simulink library "SUB_ECU_L4_MABX_HW_Interface_PIC_PB"  (R2018a)
settings: Solver=VariableStepAuto  StartTime=0.0  StopTime=10.0  RelTol=1e-3
PostLoadFcn:
  | , if any(exist('dsrtsu_mdlpostloadfcn', 'file') == [2, 3, 6]), try dsrtsu_mdlpostloadfcn('Execute', bdroot); catch fprintf('Error in PostLoadFcn (dsrtsu_mdlpostloadfcn) for model "%s":\n %s\n', bdroot, lasterr); end, end,
undefined symbols (not defined in the file or in its folder): CANR_PROPB_REAX_3_13_CHANNEL_APV, CANR_PROPB_REAX_4_13_CHANNEL_APV, CANR_PROPB_XPR_1_50_CHANNEL_APV, ENUM_CAN_RX_T, ENUM_CAN_TX_T, ENUM_REAX_OPERATION_MODE_T, ENUM_SIGNAL_HEALTH_T, ENUM_XBR_CONTROL_MODE_T, ENUM_XBR_EBI_MODE_T, ENUM_XBR_PASS_THROUGH_ACTIVE_T, ENUM_XBR_PRIORITY_T, ENUM_XPR_INHIBIT_PARK_MANUAL_T, ENUM_XPR_INHIBIT_UNPARK_MANUAL_T, ENUM_XPR_PARK_MANUAL_T, ENUM_XPR_UNPARK_MANUAL_T, PROPB_REAX_1_E4_DES_POS_SIG_SRC_APV, PROPB_REAX_1_E4_DESIRED_OPMODE_APV, PROPB_REAX_1_E4_DESIRED_POSITION_APV, PROPB_REAX_CHANNEL_APV, ptc_matlab_lib
libraries: PTC_MBDS_LIB x293, rtican x158, simulink x61, EmE_MBD_Blockset x38, rti1401lib_dio_type4 x14, simulink_need_slupdate x7, $bdroot x5, rti1401lib_adc_type4 x3, rtmapslib x3, dsa_tcpip_lib x2, SUB_ECU_L4_MABX_HW_Interface_PTC_1571 x1, rtitasklib x1
(part 20 of 49)

== system SUB_ECU_L4_MABX_HW_Interface_PIC_PB/CAN_PIC_PB/CAN_RX_VI_00/Decode_VI ==
  RawData : Inport  OutDataTypeStr=uint8  PortDimensions=17
  Add : Sum  Inputs=+  InputSameDT=on
  Add1 : Sum  Inputs=+  InputSameDT=on
  Bus Creator : BusCreator  Inputs=3
  Compare To Zero1 : simulink/Logic and Bit Operations/Compare To Zero  relop===  OutDataTypeStr=boolean
  Compare To Zero2 : simulink/Logic and Bit Operations/Compare To Zero  relop===  OutDataTypeStr=boolean
  Constant : Constant  Value=false
  Constant1 : Constant  Value=false
  Data Type Conversion{,1..16} (17 alike) : DataTypeConversion  OutDataTypeStr=uint8
  Demux : Demux  Outputs=17
  Logical Operator : Logic  OutDataTypeStr=boolean
  Logical Operator1 : Logic  OutDataTypeStr=boolean
  Mux : Mux  Inputs=17
  Relational Operator1 : RelationalOperator  Operator=~=  OutDataTypeStr=boolean  RndMeth=Nearest  InputSameDT=on
  Relational Operator2 : RelationalOperator  Operator=~=  OutDataTypeStr=boolean  RndMeth=Nearest  InputSameDT=on
  SR flip-flop : EmE_MBD_Blockset/Logic and Bit Operations/SR flip-flop
      settings: SourceProductName=PACCAR EmE MBD Blockset
  SR flip-flop1 : EmE_MBD_Blockset/Logic and Bit Operations/SR flip-flop
      settings: SourceProductName=PACCAR EmE MBD Blockset
  TRUCK_1571_VIN_CPV : Constant  Value=uint8('1XPBDP9XXGD305352')
  TRUCK_166_VIN_CPV : Constant  Value=uint8('1XKYDP9X1EJ388961')
  Unit_Delay{,1..3} (4 alike) : UnitDelay  InitialCondition=true  SampleTime=-1
      settings: AttributesFormatString=IC: %<vinit>
  VI : Outport
  wires:
  RawData/1 -> Demux/1
  Mux/1 -> Relational Operator2/2, Relational Operator1/2, Bus Creator/1  "SPN237_VehicleIdentificationNumber"
  Data Type Conversion16/1 -> Mux/17
  Data Type Conversion5/1 -> Mux/6
  Data Type Conversion/1 -> Mux/1
  Data Type Conversion1/1 -> Mux/2
  Data Type Conversion6/1 -> Mux/7
  Data Type Conversion10/1 -> Mux/11
  Data Type Conversion11/1 -> Mux/12
  Data Type Conversion7/1 -> Mux/8
  Data Type Conversion12/1 -> Mux/13
  Data Type Conversion13/1 -> Mux/15
  Data Type Conversion8/1 -> Mux/9
  Data Type Conversion15/1 -> Mux/16
  Data Type Conversion2/1 -> Mux/3
  Data Type Conversion3/1 -> Mux/4
  Data Type Conversion9/1 -> Mux/10
  Data Type Conversion4/1 -> Mux/5
  Data Type Conversion14/1 -> Mux/14
  Relational Operator1/1 -> Add/1
  Add/1 -> Compare To Zero1/1
  TRUCK_166_VIN_CPV/1 -> Relational Operator2/1
  TRUCK_1571_VIN_CPV/1 -> Relational Operator1/1
  Relational Operator2/1 -> Add1/1
  Add1/1 -> Compare To Zero2/1
  SR flip-flop/1 -> Bus Creator/3  "F_Truck1571_VIN_Match"
  SR flip-flop1/1 -> Bus Creator/2  "F_Truck166_VIN_Match"
  Demux/8 -> Data Type Conversion7/1  "byte7"
  Demux/9 -> Data Type Conversion8/1  "byte8"
  Demux/7 -> Data Type Conversion6/1  "byte6"
  Demux/6 -> Data Type Conversion5/1  "byte5"
  Demux/10 -> Data Type Conversion9/1  "byte9"
  Demux/11 -> Data Type Conversion10/1  "byte10"
  Demux/5 -> Data Type Conversion4/1  "byte4"
  Demux/12 -> Data Type Conversion11/1  "byte11"
  Demux/4 -> Data Type Conversion3/1  "byte3"
  Demux/13 -> Data Type Conversion12/1  "byte12"
  Demux/3 -> Data Type Conversion2/1  "byte2"
  Demux/2 -> Data Type Conversion1/1  "byte1"
  Demux/14 -> Data Type Conversion14/1  "byte13"
  Demux/15 -> Data Type Conversion13/1  "byte14"
  Demux/1 -> Data Type Conversion/1  "byte0"
  Demux/16 -> Data Type Conversion15/1  "byte15"
  Demux/17 -> Data Type Conversion16/1  "byte16"
  Bus Creator/1 -> VI/1  "Signals"
  Unit_Delay/1 -> SR flip-flop/2
  Constant/1 -> Unit_Delay/1
  Compare To Zero1/1 -> Logical Operator/2
  Unit_Delay1/1 -> SR flip-flop1/2
  Constant1/1 -> Unit_Delay1/1
  SR flip-flop1/2 -> Unit_Delay3/1
  Logical Operator/1 -> SR flip-flop/1
  Logical Operator1/1 -> SR flip-flop1/1
  Compare To Zero2/1 -> Logical Operator1/2
  SR flip-flop/2 -> Unit_Delay2/1
  Unit_Delay2/1 -> Logical Operator1/1
  Unit_Delay3/1 -> Logical Operator/1

== system SUB_ECU_L4_MABX_HW_Interface_PIC_PB/CAN_PIC_PB/Decode_PropB_REAX_3/decode_byte1 ==
  byte1 : Inport
  AND1 : PTC_MBDS_LIB/MBDS Standard Library/Basic Operations/Logic and Bit Operations/AND  BitwiseMode=on  Inputs=1  UseBitMask=on  BitMask=bin2dec('11110000')  OutDataTypeStr=uint8  PTC_MBDS_BlockVersion=5.41  PTC_BlockType=PTC_MBDS_AND
      settings: AttributesFormatString=bitwise  SourceProductName=PACCAR Technical Center MBDS Library
  AND2 : PTC_MBDS_LIB/MBDS Standard Library/Basic Operations/Logic and Bit Operations/AND  BitwiseMode=on  Inputs=1  UseBitMask=on  BitMask=bin2dec('00001111')  OutDataTypeStr=uint8  PTC_MBDS_BlockVersion=5.41  PTC_BlockType=PTC_MBDS_AND
      settings: AttributesFormatString=bitwise  SourceProductName=PACCAR Technical Center MBDS Library
  Bus Creator : BusCreator  Inputs=2
  "Shift_Arithmetic " : ArithShift  BitShiftNumber=4
  Out : Outport
  wires:
  "Shift_Arithmetic "/1 -> Bus Creator/2  "PropB_REAX_3_ReqOperatingMode"
  byte1/1 -> AND1/1, AND2/1
  AND2/1 -> Bus Creator/1  "PropB_REAX_3_CurrentOperatingMode"
  AND1/1 -> "Shift_Arithmetic "/1
  Bus Creator/1 -> Out/1

== system SUB_ECU_L4_MABX_HW_Interface_PIC_PB/CAN_PIC_PB/Decode_PropB_REAX_3/decode_byte2 ==
  byte2 : Inport
  Bus Creator : BusCreator  Inputs=1
  Out : Outport
  wires:
  byte2/1 -> Bus Creator/1  "PropB_REAX_3_StatusErrMsg"
  Bus Creator/1 -> Out/1

== system SUB_ECU_L4_MABX_HW_Interface_PIC_PB/CAN_PIC_PB/Decode_PropB_REAX_3/decode_byte3_byte4 ==
  byte3 : Inport
  byte4 : Inport  Port=2
  Bus Creator : BusCreator  Inputs=1
  Constant : Constant  Value=1/1024
  Data Type Conversion1 : DataTypeConversion  OutDataTypeStr=uint16  SaturateOnIntegerOverflow=on
  Data Type Conversion2 : DataTypeConversion  OutDataTypeStr=uint16  SaturateOnIntegerOverflow=on
  Data Type Conversion3 : DataTypeConversion  OutDataTypeStr=int16  ConvertRealWorld=Stored Integer (SI)
  Data Type Conversion4 : DataTypeConversion  SaturateOnIntegerOverflow=on
  OR : PTC_MBDS_LIB/MBDS Standard Library/Basic Operations/Logic and Bit Operations/OR  BitwiseMode=on  Inputs=2  UseBitMask=off  BitMask='A7'  OutDataTypeStr=uint16  PTC_MBDS_BlockVersion=5.41  PTC_BlockType=PTC_MBDS_OR
      settings: AttributesFormatString=bitwise  SourceProductName=PACCAR Technical Center MBDS Library
  Product : Product  Inputs=**  OutDataTypeStr=single  SaturateOnIntegerOverflow=on  InputSameDT=on
      settings: AttributesFormatString=Saturate: %<SaturateOnIntegerOverflow>
  Shift_Arithmetic 1 : ArithShift  BitShiftNumber=-8
  Out : Outport
  wires:
  Product/1 -> Bus Creator/1  "PropB_REAX_3_HandwheelTorque"
  Constant/1 -> Product/2
  Data Type Conversion3/1 -> Data Type Conversion4/1
  byte3/1 -> Data Type Conversion1/1
  byte4/1 -> Data Type Conversion2/1
  Data Type Conversion2/1 -> Shift_Arithmetic 1/1
  Data Type Conversion1/1 -> OR/1
  Shift_Arithmetic 1/1 -> OR/2
  OR/1 -> Data Type Conversion3/1
  Data Type Conversion4/1 -> Product/1
  Bus Creator/1 -> Out/1

== system SUB_ECU_L4_MABX_HW_Interface_PIC_PB/CAN_PIC_PB/Decode_PropB_REAX_3/decode_byte5_byte6 ==
  byte5 : Inport
  byte6 : Inport  Port=2
  Bus Creator : BusCreator  Inputs=1
  Constant1 : Constant  Value=1/1024
  Data Type Conversion1 : DataTypeConversion  SaturateOnIntegerOverflow=on
  Data Type Conversion4 : DataTypeConversion  OutDataTypeStr=uint16  SaturateOnIntegerOverflow=on
  Data Type Conversion5 : DataTypeConversion  OutDataTypeStr=uint16  SaturateOnIntegerOverflow=on
  Data Type Conversion6 : DataTypeConversion  OutDataTypeStr=int16  ConvertRealWorld=Stored Integer (SI)
  OR1 : PTC_MBDS_LIB/MBDS Standard Library/Basic Operations/Logic and Bit Operations/OR  BitwiseMode=on  Inputs=2  UseBitMask=off  BitMask='A7'  OutDataTypeStr=uint16  PTC_MBDS_BlockVersion=5.41  PTC_BlockType=PTC_MBDS_OR
      settings: AttributesFormatString=bitwise  SourceProductName=PACCAR Technical Center MBDS Library
  Product1 : Product  Inputs=**  OutDataTypeStr=single  SaturateOnIntegerOverflow=on  InputSameDT=on
      settings: AttributesFormatString=Saturate: %<SaturateOnIntegerOverflow>
  Shift_Arithmetic 2 : ArithShift  BitShiftNumber=-8
  Out : Outport
  wires:
  byte5/1 -> Data Type Conversion4/1
  byte6/1 -> Data Type Conversion5/1
  Shift_Arithmetic 2/1 -> OR1/2
  Data Type Conversion5/1 -> Shift_Arithmetic 2/1
  Data Type Conversion4/1 -> OR1/1
  OR1/1 -> Data Type Conversion6/1
  Data Type Conversion6/1 -> Data Type Conversion1/1
  Constant1/1 -> Product1/2
  Product1/1 -> Bus Creator/1  "PropB_REAX_3_HandwheelVelocity"
  Data Type Conversion1/1 -> Product1/1
  Bus Creator/1 -> Out/1

== system SUB_ECU_L4_MABX_HW_Interface_PIC_PB/CAN_PIC_PB/Decode_PropB_REAX_3/decode_byte7_byte8 ==
  byte7 : Inport
  byte8 : Inport  Port=2
  Bus Creator : BusCreator  Inputs=1
  Constant2 : Constant  Value=360/8192
  Data Type Conversion1 : DataTypeConversion  SaturateOnIntegerOverflow=on
  Data Type Conversion7 : DataTypeConversion  OutDataTypeStr=uint16  SaturateOnIntegerOverflow=on
  Data Type Conversion8 : DataTypeConversion  OutDataTypeStr=uint16  SaturateOnIntegerOverflow=on
  Data Type Conversion9 : DataTypeConversion  OutDataTypeStr=int16  ConvertRealWorld=Stored Integer (SI)
  OR2 : PTC_MBDS_LIB/MBDS Standard Library/Basic Operations/Logic and Bit Operations/OR  BitwiseMode=on  Inputs=2  UseBitMask=off  BitMask='A7'  OutDataTypeStr=uint16  PTC_MBDS_BlockVersion=5.41  PTC_BlockType=PTC_MBDS_OR
      settings: AttributesFormatString=bitwise  SourceProductName=PACCAR Technical Center MBDS Library
  Product2 : Product  Inputs=**  OutDataTypeStr=single  SaturateOnIntegerOverflow=on  InputSameDT=on
      settings: AttributesFormatString=Saturate: %<SaturateOnIntegerOverflow>
  Shift_Arithmetic 3 : ArithShift  BitShiftNumber=-8
  Out : Outport
  wires:
  byte8/1 -> Data Type Conversion8/1
  Product2/1 -> Bus Creator/1  "PropB_REAX_3_PullCompensation"
  byte7/1 -> Data Type Conversion7/1
  Data Type Conversion8/1 -> Shift_Arithmetic 3/1
  Data Type Conversion7/1 -> OR2/1
  Shift_Arithmetic 3/1 -> OR2/2
  OR2/1 -> Data Type Conversion9/1
  Constant2/1 -> Product2/2
  Data Type Conversion9/1 -> Data Type Conversion1/1
  Data Type Conversion1/1 -> Product2/1
  Bus Creator/1 -> Out/1

== system SUB_ECU_L4_MABX_HW_Interface_PIC_PB/CAN_PIC_PB/Decode_PropB_REAX_4/decode_byte1 ==
  byte1 : Inport
  AND : PTC_MBDS_LIB/MBDS Standard Library/Basic Operations/Logic and Bit Operations/AND  BitwiseMode=on  Inputs=1  UseBitMask=on  BitMask=bin2dec('00000001')  OutDataTypeStr=boolean  PTC_MBDS_BlockVersion=5.41  PTC_BlockType=PTC_MBDS_AND
      settings: AttributesFormatString=bitwise  SourceProductName=PACCAR Technical Center MBDS Library
  AND1 : PTC_MBDS_LIB/MBDS Standard Library/Basic Operations/Logic and Bit Operations/AND  BitwiseMode=on  Inputs=1  UseBitMask=on  BitMask=bin2dec('00000010')  OutDataTypeStr=uint8  PTC_MBDS_BlockVersion=5.41  PTC_BlockType=PTC_MBDS_AND
      settings: AttributesFormatString=bitwise  SourceProductName=PACCAR Technical Center MBDS Library
  AND2 : PTC_MBDS_LIB/MBDS Standard Library/Basic Operations/Logic and Bit Operations/AND  BitwiseMode=on  Inputs=1  UseBitMask=on  BitMask=bin2dec('00000100')  OutDataTypeStr=uint8  PTC_MBDS_BlockVersion=5.41  PTC_BlockType=PTC_MBDS_AND
      settings: AttributesFormatString=bitwise  SourceProductName=PACCAR Technical Center MBDS Library
  Bus Creator : BusCreator  Inputs=3
  Data Type Conversion : DataTypeConversion  OutDataTypeStr=boolean  SaturateOnIntegerOverflow=on
  Data Type Conversion1 : DataTypeConversion  OutDataTypeStr=boolean  SaturateOnIntegerOverflow=on
  "Shift_Arithmetic " : ArithShift  BitShiftNumber=1
  Shift_Arithmetic 1 : ArithShift  BitShiftNumber=2
  Out : Outport
  wires:
  AND/1 -> Bus Creator/1  "PropB_REAX_4_AbsSteeringPosValid"
  AND2/1 -> Shift_Arithmetic 1/1
  byte1/1 -> AND2/1, AND1/1, AND/1
  AND1/1 -> "Shift_Arithmetic "/1
  "Shift_Arithmetic "/1 -> Data Type Conversion/1
  Shift_Arithmetic 1/1 -> Data Type Conversion1/1
  Bus Creator/1 -> Out/1
  Data Type Conversion/1 -> Bus Creator/2  "PropB_REAX_4_PositionIndexValid"
  Data Type Conversion1/1 -> Bus Creator/3  "PropB_REAX_4_DriverControlledEffortsEnabled"

== system SUB_ECU_L4_MABX_HW_Interface_PIC_PB/CAN_PIC_PB/Decode_PropB_REAX_4/decode_byte2 ==
  byte2 : Inport
  Bus Creator : BusCreator  Inputs=1
  SignalConversion : SignalConversion  ConversionOutput=Contiguous copy  OverrideOpt=off
  Out : Outport
  wires:
  byte2/1 -> SignalConversion/1
  SignalConversion/1 -> Bus Creator/1  "PropB_REAX_4_ControlOperatingMode"
  Bus Creator/1 -> Out/1

== system SUB_ECU_L4_MABX_HW_Interface_PIC_PB/CAN_PIC_PB/Decode_PropB_REAX_4/decode_byte3 ==
  byte3 : Inport
  Bus Creator : BusCreator  Inputs=1
  SignalConversion : SignalConversion  ConversionOutput=Contiguous copy  OverrideOpt=off
  Out : Outport
  wires:
  byte3/1 -> SignalConversion/1
  SignalConversion/1 -> Bus Creator/1  "PropB_REAX_4_SystemMode"
  Bus Creator/1 -> Out/1

== system SUB_ECU_L4_MABX_HW_Interface_PIC_PB/CAN_PIC_PB/Decode_PropB_REAX_4/decode_byte5 ==
  byte5 : Inport
  Bus Creator : BusCreator  Inputs=1
  Data Type Conversion4 : DataTypeConversion  OutDataTypeStr=int8  ConvertRealWorld=Stored Integer (SI)
  Data Type Conversion5 : DataTypeConversion  OutDataTypeStr=double  SaturateOnIntegerOverflow=on
  Out : Outport
  wires:
  byte5/1 -> Data Type Conversion4/1
  Data Type Conversion4/1 -> Data Type Conversion5/1
  Data Type Conversion5/1 -> Bus Creator/1  "PropB_REAX_4_PercHandwheelTorque"
  Bus Creator/1 -> Out/1

== system SUB_ECU_L4_MABX_HW_Interface_PIC_PB/CAN_PIC_PB/Decode_PropB_REAX_4/decode_byte6_byte7 ==
  byte6 : Inport
  byte7 : Inport  Port=2
  Bus Creator : BusCreator  Inputs=1
  Data Type Conversion6 : DataTypeConversion  OutDataTypeStr=uint16  SaturateOnIntegerOverflow=on
  Data Type Conversion7 : DataTypeConversion  OutDataTypeStr=uint16  SaturateOnIntegerOverflow=on
  Data Type Conversion8 : DataTypeConversion  OutDataTypeStr=int16  ConvertRealWorld=Stored Integer (SI)
  Data Type Conversion9 : DataTypeConversion  OutDataTypeStr=double  SaturateOnIntegerOverflow=on
  OR : PTC_MBDS_LIB/MBDS Standard Library/Basic Operations/Logic and Bit Operations/OR  BitwiseMode=on  Inputs=2  UseBitMask=off  BitMask='A7'  OutDataTypeStr=uint16  PTC_MBDS_BlockVersion=5.41  PTC_BlockType=PTC_MBDS_OR
      settings: AttributesFormatString=bitwise  SourceProductName=PACCAR Technical Center MBDS Library
  Shift_Arithmetic 2 : ArithShift  BitShiftNumber=-8
  Out : Outport
  wires:
  Data Type Conversion9/1 -> Bus Creator/1  "PropB_REAX_4_AbsSteeringAngle"
  byte6/1 -> Data Type Conversion6/1
  byte7/1 -> Data Type Conversion7/1
  Data Type Conversion6/1 -> OR/1
  Data Type Conversion7/1 -> Shift_Arithmetic 2/1
  Shift_Arithmetic 2/1 -> OR/2
  Data Type Conversion8/1 -> Data Type Conversion9/1
  OR/1 -> Data Type Conversion8/1
  Bus Creator/1 -> Out/1

== system SUB_ECU_L4_MABX_HW_Interface_PIC_PB/CAN_PIC_PB/Decode_PropB_REAX_4/decode_byte8 ==
  byte8 : Inport
  Bus Creator : BusCreator  Inputs=1
  Data Type Conversion10 : DataTypeConversion  OutDataTypeStr=int8  ConvertRealWorld=Stored Integer (SI)
  Data Type Conversion11 : DataTypeConversion  OutDataTypeStr=double  SaturateOnIntegerOverflow=on
  Out : Outport
  wires:
  Data Type Conversion11/1 -> Bus Creator/1  "PropB_REAX_4_PercMotorTorque"
  Data Type Conversion10/1 -> Data Type Conversion11/1
  byte8/1 -> Data Type Conversion10/1
  Bus Creator/1 -> Out/1

== system SUB_ECU_L4_MABX_HW_Interface_PIC_PB/DIGITAL/Debounce/On Delay ==
  In : Inport
  time_ms : Inport  Port=2
  AND : Logic  IconShape=distinctive  AllPortsSameDT=off  OutDataTypeStr=boolean
  Compare To Zero : simulink/Logic and Bit Operations/Compare To Zero  relop=>  OutDataTypeStr=boolean
  Constant0 : Constant  Value=0
  Constant1 : Constant
  Gain : Gain  Gain=0.1
  LessThanOrEqual : RelationalOperator  Operator=<=  OutDataTypeStr=boolean  RndMeth=Simplest
  OR1 : Logic  Operator=OR  IconShape=distinctive  AllPortsSameDT=off  OutDataTypeStr=boolean
  Sum : Sum  Inputs=++|
  Switch : Switch  Criteria=u2 > Threshold
  Unit Delay : UnitDelay  SampleTime=-1
  Unit Delay1 : UnitDelay  SampleTime=-1
  out : Outport
  wires:
  Switch/1 -> LessThanOrEqual/1, Unit Delay/1, Compare To Zero/1
  AND/1 -> out/1, Unit Delay1/1
  Compare To Zero/1 -> AND/1
  LessThanOrEqual/1 -> AND/2
  Sum/1 -> Switch/1
  Unit Delay1/1 -> OR1/2
  In/1 -> OR1/1
  Constant0/1 -> Switch/3
  OR1/1 -> Switch/2
  Unit Delay/1 -> Sum/1
  Constant1/1 -> Sum/2
  Gain/1 -> LessThanOrEqual/2
  time_ms/1 -> Gain/1

== system SUB_ECU_L4_MABX_HW_Interface_PIC_PB/DIGITAL/PWM pedal input management/Determine common angle ==
  Pedal_1_pwm_health_state : Inport
  F_Pedal_pwm_sens_total_failure : Inport  Port=2
  Pedal_2_pwm_health_state : Inport  Port=3
  Pedal_1_pwm_angle_arbitrated : Inport  Port=4
  Pedal_2_pwm_angle_arbitrated : Inport  Port=5
  DEFAULT_VALUE : Inport  Port=6
  Compare To Constant1 : simulink/Logic and Bit Operations/Compare To Constant  relop===  const=ENUM_SIGNAL_HEALTH_T.FAULT_ACTIVE  OutDataTypeStr=boolean
  Compare To Constant3 : simulink/Logic and Bit Operations/Compare To Constant  relop===  const=ENUM_SIGNAL_HEALTH_T.FAULT_ACTIVE  OutDataTypeStr=boolean
  If_Then_Else : EmE_MBD_Blockset/Signal Routing/If_Then_Else
      settings: SourceProductName=PACCAR EmE MBD Blockset
  If_Then_Else1 : EmE_MBD_Blockset/Signal Routing/If_Then_Else
      settings: SourceProductName=PACCAR EmE MBD Blockset
  If_Then_Else2 : EmE_MBD_Blockset/Signal Routing/If_Then_Else
      settings: SourceProductName=PACCAR EmE MBD Blockset
  MinMax : MinMax  Inputs=2  InputSameDT=on
  Pedal_pwm_angle_common : Outport
  wires:
  MinMax/1 -> If_Then_Else/3
  If_Then_Else1/1 -> MinMax/1  "Pedal_1_pwm_corr"
  If_Then_Else2/1 -> MinMax/2  "Pedal_2_pwm_corr"
  Compare To Constant1/1 -> If_Then_Else2/1
  Pedal_1_pwm_angle_arbitrated/1 -> If_Then_Else1/3, If_Then_Else2/2
  Compare To Constant3/1 -> If_Then_Else1/1
  Pedal_2_pwm_health_state/1 -> Compare To Constant1/1
  Pedal_1_pwm_health_state/1 -> Compare To Constant3/1
  If_Then_Else/1 -> Pedal_pwm_angle_common/1  "Pedal_pwm_angle_common"
  DEFAULT_VALUE/1 -> If_Then_Else/2
  Pedal_2_pwm_angle_arbitrated/1 -> If_Then_Else1/2, If_Then_Else2/3
  F_Pedal_pwm_sens_total_failure/1 -> If_Then_Else/1

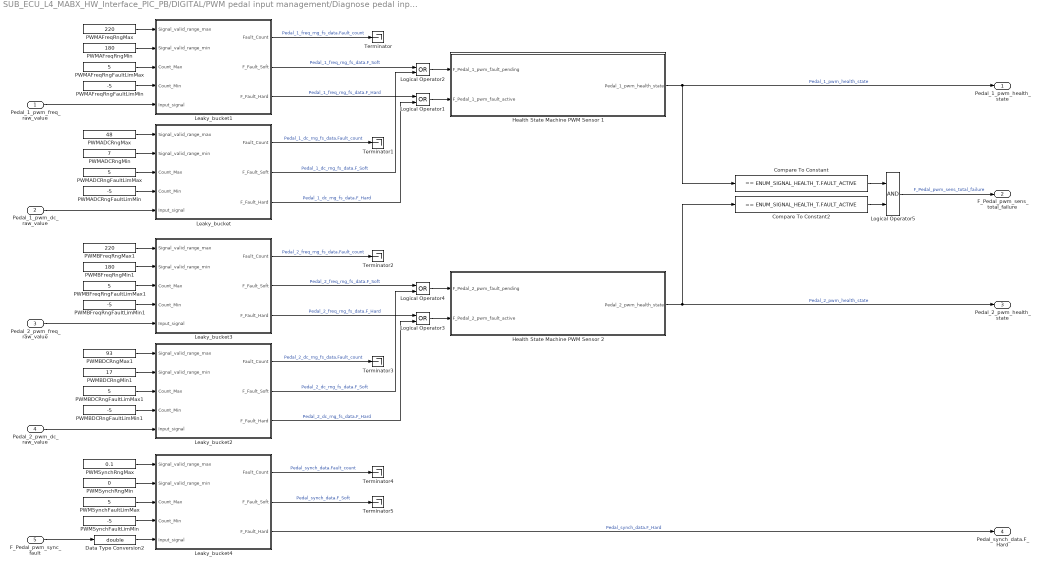
== system SUB_ECU_L4_MABX_HW_Interface_PIC_PB/DIGITAL/PWM pedal input management/Diagnose pedal input signals ==
  Pedal_1_pwm_freq_raw_value : Inport
  Pedal_1_pwm_dc_raw_value : Inport  Port=2
  Pedal_2_pwm_freq_raw_value : Inport  Port=3
  Pedal_2_pwm_dc_raw_value : Inport  Port=4
  F_Pedal_pwm_sync_fault : Inport  Port=5
  Compare To Constant : simulink/Logic and Bit Operations/Compare To Constant  relop===  const=ENUM_SIGNAL_HEALTH_T.FAULT_ACTIVE  OutDataTypeStr=boolean
  Compare To Constant2 : simulink/Logic and Bit Operations/Compare To Constant  relop===  const=ENUM_SIGNAL_HEALTH_T.FAULT_ACTIVE  OutDataTypeStr=boolean
  Data Type Conversion2 : DataTypeConversion  OutDataTypeStr=double  SaturateOnIntegerOverflow=on
  Health State Machine PWM Sensor 1 : Stateflow chart  TreatAsAtomicUnit=on
  Health State Machine PWM Sensor 2 : Stateflow chart  TreatAsAtomicUnit=on
  Leaky_bucket : Subsystem
  Leaky_bucket1 : Subsystem
  Leaky_bucket2 : Subsystem
  Leaky_bucket3 : Subsystem
  Leaky_bucket4 : Subsystem
  Logical Operator{1..4} (4 alike) : Logic  Operator=OR  OutDataTypeStr=boolean
  Logical Operator5 : Logic  OutDataTypeStr=boolean
  PWMADCRngFaultLimMax : Constant  Value=5
  PWMADCRngFaultLimMin : Constant  Value=-5
  PWMADCRngMax : Constant  Value=48
  PWMADCRngMin : Constant  Value=7
  PWMAFreqRngFaultLimMax : Constant  Value=5
  PWMAFreqRngFaultLimMin : Constant  Value=-5
  PWMAFreqRngMax : Constant  Value=220
  PWMAFreqRngMin : Constant  Value=180
  PWMBDCRngFaultLimMax1 : Constant  Value=5
  PWMBDCRngFaultLimMin1 : Constant  Value=-5
  PWMBDCRngMax1 : Constant  Value=93
  PWMBDCRngMin1 : Constant  Value=17
  PWMBFreqRngFaultLimMax1 : Constant  Value=5
  PWMBFreqRngFaultLimMin1 : Constant  Value=-5
  PWMBFreqRngMax1 : Constant  Value=220
  PWMBFreqRngMin1 : Constant  Value=180
  PWMSynchFaultLimMax : Constant  Value=5
  PWMSynchFaultLimMin : Constant  Value=-5
  PWMSynchRngMax : Constant  Value=0.1
  PWMSynchRngMin : Constant  Value=0
  Terminator{,1..5} (6 alike) : Terminator
  Pedal_1_pwm_health_state : Outport
  F_Pedal_pwm_sens_total_failure : Outport  Port=2
  Pedal_2_pwm_health_state : Outport  Port=3
  Pedal_synch_data.F_Hard : Outport  Port=4
  wires:
  Pedal_2_pwm_dc_raw_value/1 -> Leaky_bucket2/5(Input_signal)
  Pedal_2_pwm_freq_raw_value/1 -> Leaky_bucket3/5(Input_signal)
  Pedal_1_pwm_dc_raw_value/1 -> Leaky_bucket/5(Input_signal)
  Leaky_bucket4/2(F_Fault_Soft) -> Terminator5/1  "Pedal_synch_data.F_Soft"
  Leaky_bucket4/1(Fault_Count) -> Terminator4/1  "Pedal_synch_data.Fault_count"
  Leaky_bucket4/3(F_Fault_Hard) -> Pedal_synch_data.F_Hard/1  "Pedal_synch_data.F_Hard"
  PWMSynchFaultLimMin/1 -> Leaky_bucket4/4(Count_Min)
  F_Pedal_pwm_sync_fault/1 -> Data Type Conversion2/1
  PWMSynchFaultLimMax/1 -> Leaky_bucket4/3(Count_Max)
  PWMSynchRngMin/1 -> Leaky_bucket4/2(Signal_valid_range_min)
  PWMSynchRngMax/1 -> Leaky_bucket4/1(Signal_valid_range_max)
  Logical Operator5/1 -> F_Pedal_pwm_sens_total_failure/1  "F_Pedal_pwm_sens_total_failure"
  Compare To Constant2/1 -> Logical Operator5/2
  Compare To Constant/1 -> Logical Operator5/1
  Health State Machine PWM Sensor 1/1(Pedal_1_pwm_health_state) -> Compare To Constant/1, Pedal_1_pwm_health_state/1  "Pedal_1_pwm_health_state"
  Logical Operator4/1 -> Health State Machine PWM Sensor 2/1(F_Pedal_2_pwm_fault_pending)
  Logical Operator3/1 -> Health State Machine PWM Sensor 2/2(F_Pedal_2_pwm_fault_active)
  Leaky_bucket3/1(Fault_Count) -> Terminator2/1  "Pedal_2_freq_rng_fs_data.Fault_count"
  PWMBFreqRngFaultLimMin1/1 -> Leaky_bucket3/4(Count_Min)
  PWMBFreqRngFaultLimMax1/1 -> Leaky_bucket3/3(Count_Max)
  PWMBFreqRngMax1/1 -> Leaky_bucket3/1(Signal_valid_range_max)
  PWMBFreqRngMin1/1 -> Leaky_bucket3/2(Signal_valid_range_min)
  Leaky_bucket2/2(F_Fault_Soft) -> Logical Operator4/2  "Pedal_2_dc_rng_fs_data.F_Soft"
  Leaky_bucket2/1(Fault_Count) -> Terminator3/1  "Pedal_2_dc_rng_fs_data.Fault_count"
  Leaky_bucket2/3(F_Fault_Hard) -> Logical Operator3/2  "Pedal_2_dc_rng_fs_data.F_Hard"
  PWMBDCRngFaultLimMin1/1 -> Leaky_bucket2/4(Count_Min)
  PWMBDCRngFaultLimMax1/1 -> Leaky_bucket2/3(Count_Max)
  PWMBDCRngMin1/1 -> Leaky_bucket2/2(Signal_valid_range_min)
  PWMBDCRngMax1/1 -> Leaky_bucket2/1(Signal_valid_range_max)
  Health State Machine PWM Sensor 2/1(Pedal_2_pwm_health_state) -> Compare To Constant2/1, Pedal_2_pwm_health_state/1  "Pedal_2_pwm_health_state"
  Leaky_bucket3/2(F_Fault_Soft) -> Logical Operator4/1  "Pedal_2_freq_rng_fs_data.F_Soft"
  Leaky_bucket3/3(F_Fault_Hard) -> Logical Operator3/1  "Pedal_2_freq_rng_fs_data.F_Hard"
  Logical Operator2/1 -> Health State Machine PWM Sensor 1/1(F_Pedal_1_pwm_fault_pending)
  Logical Operator1/1 -> Health State Machine PWM Sensor 1/2(F_Pedal_1_pwm_fault_active)
  Leaky_bucket1/1(Fault_Count) -> Terminator/1  "Pedal_1_freq_rng_fs_data.Fault_count"
  PWMAFreqRngFaultLimMin/1 -> Leaky_bucket1/4(Count_Min)
  PWMAFreqRngFaultLimMax/1 -> Leaky_bucket1/3(Count_Max)
  PWMAFreqRngMax/1 -> Leaky_bucket1/1(Signal_valid_range_max)
  PWMAFreqRngMin/1 -> Leaky_bucket1/2(Signal_valid_range_min)
  Leaky_bucket/2(F_Fault_Soft) -> Logical Operator2/2  "Pedal_1_dc_rng_fs_data.F_Soft"
  Leaky_bucket/1(Fault_Count) -> Terminator1/1  "Pedal_1_dc_rng_fs_data.Fault_count"
  Leaky_bucket/3(F_Fault_Hard) -> Logical Operator1/2  "Pedal_1_dc_rng_fs_data.F_Hard"
  PWMADCRngFaultLimMin/1 -> Leaky_bucket/4(Count_Min)
  PWMADCRngFaultLimMax/1 -> Leaky_bucket/3(Count_Max)
  PWMADCRngMin/1 -> Leaky_bucket/2(Signal_valid_range_min)
  PWMADCRngMax/1 -> Leaky_bucket/1(Signal_valid_range_max)
  Leaky_bucket1/2(F_Fault_Soft) -> Logical Operator2/1  "Pedal_1_freq_rng_fs_data.F_Soft"
  Leaky_bucket1/3(F_Fault_Hard) -> Logical Operator1/1  "Pedal_1_freq_rng_fs_data.F_Hard"
  Data Type Conversion2/1 -> Leaky_bucket4/5(Input_signal)
  Pedal_1_pwm_freq_raw_value/1 -> Leaky_bucket1/5(Input_signal)

== system SUB_ECU_L4_MABX_HW_Interface_PIC_PB/DIGITAL/PWM pedal input management/Fault arbitration ==
  Pedal_1_pwm_health_state : Inport
  Pedal_1_pwm_undefault : Inport  Port=2
  DEFAULT_VALUE : Inport  Port=3
  Pedal_2_pwm_health_state : Inport  Port=4
  Pedal_2_pwm_undefault : Inport  Port=5
  Compare To Constant1 : simulink/Logic and Bit Operations/Compare To Constant  relop===  const=ENUM_SIGNAL_HEALTH_T.FAULT_PENDING  OutDataTypeStr=boolean
  Compare To Constant3 : simulink/Logic and Bit Operations/Compare To Constant  relop===  const=ENUM_SIGNAL_HEALTH_T.FAULT_ACTIVE  OutDataTypeStr=boolean
  Compare To Constant4 : simulink/Logic and Bit Operations/Compare To Constant  relop===  const=ENUM_SIGNAL_HEALTH_T.FAULT_PENDING  OutDataTypeStr=boolean
  Compare To Constant5 : simulink/Logic and Bit Operations/Compare To Constant  relop===  const=ENUM_SIGNAL_HEALTH_T.FAULT_ACTIVE  OutDataTypeStr=boolean
  If_Then_Else{,1..3} (4 alike) : EmE_MBD_Blockset/Signal Routing/If_Then_Else
      settings: SourceProductName=PACCAR EmE MBD Blockset
  Logical Operator{5..8} (4 alike) : Logic  Operator=NOT  OutDataTypeStr=boolean
  Unit Delay External IC : simulink_need_slupdate/Unit Delay External IC  tsamp=-1
      settings: SourceProductName=Simulink  SourceProductBaseCode=SL
  Unit Delay External IC1 : simulink_need_slupdate/Unit Delay External IC  tsamp=-1
      settings: SourceProductName=Simulink  SourceProductBaseCode=SL
  Pedal_1_pwm_angle_arbitrated : Outport
  Pedal_2_pwm_angle_arbitrated : Outport  Port=2
  wires:
  Compare To Constant4/1 -> Logical Operator8/1
  Logical Operator8/1 -> If_Then_Else3/1
  [DEFAULT_VALUE] -> Unit Delay External IC1/2, If_Then_Else2/3
  If_Then_Else2/1 -> Pedal_2_pwm_angle_arbitrated/1  "Pedal_2_pwm_angle_arbitrated"
  Unit Delay External IC1/1 -> If_Then_Else3/3
  Unit Delay External IC/1 -> If_Then_Else1/3
  Compare To Constant5/1 -> Logical Operator7/1
  Compare To Constant1/1 -> Logical Operator6/1
  Logical Operator5/1 -> If_Then_Else/1
  Compare To Constant3/1 -> Logical Operator5/1
  Pedal_1_pwm_health_state/1 -> Compare To Constant3/1, Compare To Constant1/1
  If_Then_Else3/1 -> If_Then_Else2/2, Unit Delay External IC1/1
  Logical Operator6/1 -> If_Then_Else1/1
  Pedal_2_pwm_health_state/1 -> Compare To Constant4/1, Compare To Constant5/1
  Pedal_2_pwm_undefault/1 -> If_Then_Else3/2
  Logical Operator7/1 -> If_Then_Else2/1
  If_Then_Else1/1 -> Unit Delay External IC/1, If_Then_Else/2
  Pedal_1_pwm_undefault/1 -> If_Then_Else1/2
  DEFAULT_VALUE/1 -> If_Then_Else/3, Unit Delay External IC/2, [DEFAULT_VALUE]
  If_Then_Else/1 -> Pedal_1_pwm_angle_arbitrated/1  "Pedal_1_pwm_angle_arbitrated"

== system SUB_ECU_L4_MABX_HW_Interface_PIC_PB/DIGITAL/PWM pedal input management/PWM signal filtering conversion ==
  Pedal _1_pwm_dc_raw_value : Inport
  Pedal _2_pwm_dc_raw_value : Inport  Port=2
  Constant : Constant  Value=false
  Constant1 : Constant  Value=false
  LPF_first_order : EmE_MBD_Blockset/Discrete/LPF_first_order
      settings: SourceProductName=PACCAR EmE MBD Blockset
  LPF_first_order1 : EmE_MBD_Blockset/Discrete/LPF_first_order
      settings: SourceProductName=PACCAR EmE MBD Blockset
  PEDAL_PWM_ANGLE_SENS_1_MPV : Lookup_n-D  NumberOfTableDimensions=1  BreakpointsForDimension1=[0 10 20 45 90 91 99.5 100]  Table=[-25 0 28.57 100 228.57 231.43 255 255]  ExtrapMethod=Clip  UseLastTableValue=on  InputSameDT=on
      settings: AttributesFormatString=|
      | X: %<BreakpointsForDimension1>
      | Y: %<Table>
  PEDAL_PWM_ANGLE_SENS_2_MPV : Lookup_n-D  NumberOfTableDimensions=1  BreakpointsForDimension1=[0 10 20 45 90 91 99.5 100]  Table=[-25 -14.29 0 35.71 100 101.43 113.57 114.29]  ExtrapMethod=Clip  UseLastTableValue=on  InputSameDT=on
      settings: AttributesFormatString=|
      | X: %<BreakpointsForDimension1>
      | Y: %<Table>
  PEDAL_PWM_SENSOR_DATA_APV.T1_CONST : Constant  Value=0.1
  PEDAL_PWM_SENSOR_DATA_APV.T2_CONST : Constant  Value=0.1
  Unit_Delay : UnitDelay  InitialCondition=true  SampleTime=-1
      settings: AttributesFormatString=IC: %<vinit>
  Unit_Delay1 : UnitDelay  InitialCondition=true  SampleTime=-1
      settings: AttributesFormatString=IC: %<vinit>
  dT : Constant  Value=0.01
  dT1 : Constant  Value=0.01
  Pedal_1_pwm_undefault : Outport
  Pedal_2_pwm_undefault : Outport  Port=2
  wires:
  PEDAL_PWM_ANGLE_SENS_1_MPV/1 -> Pedal_1_pwm_undefault/1  "Pedal_1_pwm_undefault"
  PEDAL_PWM_ANGLE_SENS_2_MPV/1 -> Pedal_2_pwm_undefault/1  "Pedal_2_pwm_undefault"
  LPF_first_order1/1 -> PEDAL_PWM_ANGLE_SENS_2_MPV/1
  dT1/1 -> LPF_first_order1/5
  Constant1/1 -> Unit_Delay1/1
  Pedal _2_pwm_dc_raw_value/1 -> LPF_first_order1/2, LPF_first_order1/3
  PEDAL_PWM_SENSOR_DATA_APV.T2_CONST/1 -> LPF_first_order1/4
  Unit_Delay1/1 -> LPF_first_order1/1
  LPF_first_order/1 -> PEDAL_PWM_ANGLE_SENS_1_MPV/1
  dT/1 -> LPF_first_order/5
  Constant/1 -> Unit_Delay/1
  Pedal _1_pwm_dc_raw_value/1 -> LPF_first_order/3, LPF_first_order/2
  PEDAL_PWM_SENSOR_DATA_APV.T1_CONST/1 -> LPF_first_order/4
  Unit_Delay/1 -> LPF_first_order/1

== system SUB_ECU_L4_MABX_HW_Interface_PIC_PB/DIGITAL/PWM pedal input management/Synchronization check sensor 1 and 2 ==
  Pedal_pwm_angle_common : Inport
  Pedal_1_pwm_undefault : Inport  Port=2
  Pedal_2_pwm_undefault : Inport  Port=3
  Abs : Abs
  PEDAL_PWM_ANGLE_DEV_MPV : Lookup_n-D  NumberOfTableDimensions=1  BreakpointsForDimension1=[0 14 15 20 80 85 86 100]  Table=[10 10 10 10 10 10 10 10]  ExtrapMethod=Clip  UseLastTableValue=on  InputSameDT=on
      settings: AttributesFormatString=|
      | X: %<BreakpointsForDimension1>
      | Y: %<Table>
  Relational Operator : RelationalOperator  Operator=>  OutDataTypeStr=boolean  RndMeth=Nearest
  Subtract : Sum  Inputs=+-  InputSameDT=on
  F_Pedal_pwm_sync_fault : Outport
  wires:
  PEDAL_PWM_ANGLE_DEV_MPV/1 -> Relational Operator/2
  Pedal_pwm_angle_common/1 -> PEDAL_PWM_ANGLE_DEV_MPV/1
  Relational Operator/1 -> F_Pedal_pwm_sync_fault/1  "F_Pedal_pwm_sync_fault"
  Abs/1 -> Relational Operator/1
  Subtract/1 -> Abs/1
  Pedal_1_pwm_undefault/1 -> Subtract/1
  Pedal_2_pwm_undefault/1 -> Subtract/2

== system SUB_ECU_L4_MABX_HW_Interface_PIC_PB/DIGITAL/Signal Check/RationalityCheck ==
  UndefaultStatus : Inport
  Chart : Stateflow chart  TreatAsAtomicUnit=on
  DiagPassed : Outport
  wires:
  UndefaultStatus/1 -> Chart/1(Input)
  Chart/1(DiagPassed) -> DiagPassed/1

== system SUB_ECU_L4_MABX_HW_Interface_PIC_PB/ETHERNET/Data RX/RTMaps Health Check ==
  Heartbeat : Inport
  Constant : Constant
  Constant1 : Constant  Value=0
  Constant2 : Constant  Value=0  OutDataTypeStr=boolean
  Constant3 : Constant  OutDataTypeStr=boolean
  Detect Rise Positive1 : simulink/Logic and Bit Operations/Detect Rise Positive  vinit=0  OutDataTypeStr=boolean
  Sum : Sum  Inputs=|++
  Switch : Switch  Criteria=u2 > Threshold
  Switch1 : Switch  Criteria=u2 > Threshold  Threshold=100
  Unit Delay : UnitDelay  SampleTime=-1
  Status : Outport
  wires:
  Unit Delay/1 -> Sum/2
  Constant/1 -> Sum/1
  Constant2/1 -> Switch1/1
  Sum/1 -> Switch/3
  Heartbeat/1 -> Detect Rise Positive1/1
  Switch/1 -> Switch1/2, Unit Delay/1  "Count"
  Constant1/1 -> Switch/1
  Detect Rise Positive1/1 -> Switch/2
  Constant3/1 -> Switch1/3
  Switch1/1 -> Status/1  "Heartbeat_Ok"

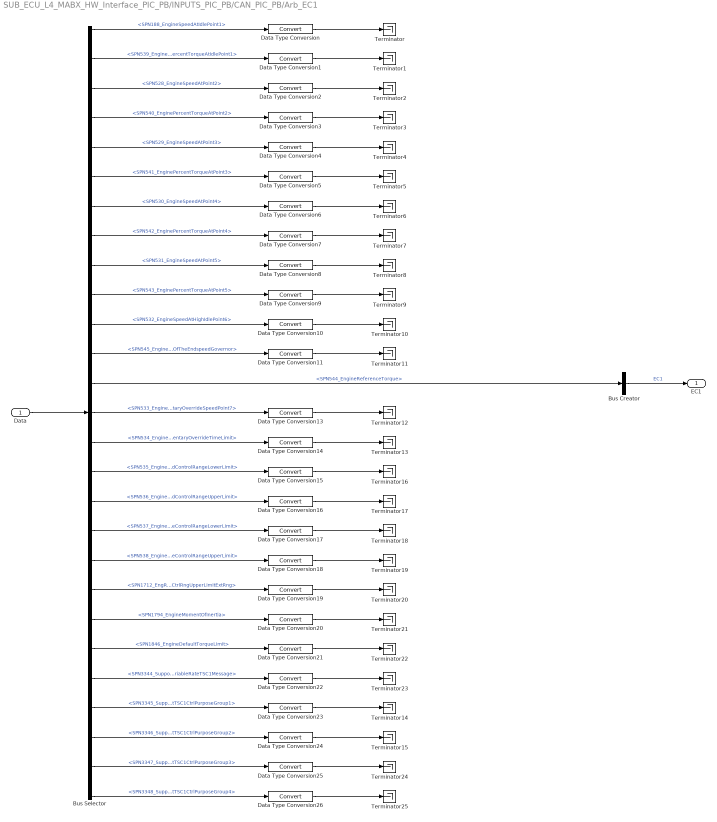
== system SUB_ECU_L4_MABX_HW_Interface_PIC_PB/INPUTS_PIC_PB/CAN_PIC_PB/Arb_EC1 ==
  Data : Inport
  Bus Creator : BusCreator  Inputs=1
  Bus Selector : BusSelector  OutputSignals=Signals.SPN188_EngineSpeedAtIdlePoint1,Signals.SPN539_EnginePercentTorqueAtIdlePoint1,Signals.SPN528_EngineSpeedAtPoint2,Signals.SPN540_EnginePercentTorqueAtPoint2,Signals.SPN529_EngineSpeedAtPoint3,Signals.SPN541_EnginePercentTorqueAtPoint3,Signals.SPN530_EngineSpeedAtPoint4,Signals.SPN542_EnginePercentTorqueAtPoint4,Signals.SPN531_EngineSpeedAtPoint5,Signals.SPN543_EnginePercentTorqueAtPoint5,Signals.SPN532_EngineSpeedAtHighIdlePoint6,Signals.SPN545_EngineGainKpOfTheEndspeedGovernor,Signals.SPN544_EngineReferenceTorque,Signals.SPN533_EngineMaximumMomentaryOverrideSpeedPoint7,Signals.SPN534_EngineMaximumMomentaryOverrideTimeLimit,Signals.SPN535_EngineRequestedSpeedControlRangeLowerLimit,Signals.SPN536_EngineRequestedSpeedControlRangeUpperLimit,Signals.SPN537_EngineRequestedTorqueControlRangeLowerLimit,Signals.SPN538_EngineRequestedTorqueControlRangeUpperLimit,Signals.SPN1712_EngRequestedSpeedCtrlRngUpperLimitExtRng,Signals.SPN1794_EngineMomentOfInertia,Signals.SPN1846_EngineDefaultTorqueLimit,Signals.SPN3344_SupportVariableRateTSC1Message,Signals.SPN3345_SupportTSC1CtrlPurposeGroup1,Signals.SPN3346_SupportTSC1CtrlPurposeGroup2,Signals.SPN3347_SupportTSC1CtrlPurposeGroup3,Signals.SPN3348_SupportTSC1CtrlPurposeGroup4
  Data Type Conversion{,1..11,13..26} (26 alike) : DataTypeConversion  SaturateOnIntegerOverflow=on
  Terminator{,1..25} (26 alike) : Terminator
      settings: InitFcn=|
      | try
      |    MBDS_BlockCallback('Update', gcb);
      | end
  EC1 : Outport
  wires:
  Bus Creator/1 -> EC1/1  "EC1"
  Data Type Conversion24/1 -> Terminator15/1
  Data Type Conversion25/1 -> Terminator24/1
  Data Type Conversion26/1 -> Terminator25/1
  Data Type Conversion19/1 -> Terminator20/1
  Data Type Conversion18/1 -> Terminator19/1
  Data Type Conversion21/1 -> Terminator22/1
  Data Type Conversion16/1 -> Terminator17/1
  Data Type Conversion17/1 -> Terminator18/1
  Data Type Conversion23/1 -> Terminator14/1
  Data Type Conversion22/1 -> Terminator23/1
  Data Type Conversion20/1 -> Terminator21/1
  Data Type Conversion11/1 -> Terminator11/1
  Data Type Conversion8/1 -> Terminator8/1
  Data Type Conversion15/1 -> Terminator16/1
  Data Type Conversion14/1 -> Terminator13/1
  Data Type Conversion13/1 -> Terminator12/1
  Data Type Conversion10/1 -> Terminator10/1
  Data Type Conversion9/1 -> Terminator9/1
  Data Type Conversion4/1 -> Terminator4/1
  Data Type Conversion7/1 -> Terminator7/1
  Data Type Conversion5/1 -> Terminator5/1
  Data Type Conversion6/1 -> Terminator6/1
  Data Type Conversion3/1 -> Terminator3/1
  Data Type Conversion2/1 -> Terminator2/1
  Data Type Conversion1/1 -> Terminator1/1
  Data Type Conversion/1 -> Terminator/1
  Bus Selector/27 -> Data Type Conversion26/1  "<SPN3348_SupportTSC1CtrlPurposeGroup4>"
  Bus Selector/26 -> Data Type Conversion25/1  "<SPN3347_SupportTSC1CtrlPurposeGroup3>"
  Bus Selector/25 -> Data Type Conversion24/1  "<SPN3346_SupportTSC1CtrlPurposeGroup2>"
  Bus Selector/24 -> Data Type Conversion23/1  "<SPN3345_SupportTSC1CtrlPurposeGroup1>"
  Bus Selector/23 -> Data Type Conversion22/1  "<SPN3344_SupportVariableRateTSC1Message>"
  Bus Selector/22 -> Data Type Conversion21/1  "<SPN1846_EngineDefaultTorqueLimit>"
  Bus Selector/21 -> Data Type Conversion20/1  "<SPN1794_EngineMomentOfInertia>"
  Bus Selector/20 -> Data Type Conversion19/1  "<SPN1712_EngRequestedSpeedCtrlRngUpperLimitExtRng>"
  Bus Selector/19 -> Data Type Conversion18/1  "<SPN538_EngineRequestedTorqueControlRangeUpperLimit>"
  Bus Selector/18 -> Data Type Conversion17/1  "<SPN537_EngineRequestedTorqueControlRangeLowerLimit>"
  Bus Selector/17 -> Data Type Conversion16/1  "<SPN536_EngineRequestedSpeedControlRangeUpperLimit>"
  Bus Selector/16 -> Data Type Conversion15/1  "<SPN535_EngineRequestedSpeedControlRangeLowerLimit>"
  Bus Selector/15 -> Data Type Conversion14/1  "<SPN534_EngineMaximumMomentaryOverrideTimeLimit>"
  Bus Selector/14 -> Data Type Conversion13/1  "<SPN533_EngineMaximumMomentaryOverrideSpeedPoint7>"
  Bus Selector/13 -> Bus Creator/1  "<SPN544_EngineReferenceTorque>"
  Bus Selector/11 -> Data Type Conversion10/1  "<SPN532_EngineSpeedAtHighIdlePoint6>"
  Bus Selector/10 -> Data Type Conversion9/1  "<SPN543_EnginePercentTorqueAtPoint5>"
  Bus Selector/9 -> Data Type Conversion8/1  "<SPN531_EngineSpeedAtPoint5>"
  Bus Selector/8 -> Data Type Conversion7/1  "<SPN542_EnginePercentTorqueAtPoint4>"
  Bus Selector/7 -> Data Type Conversion6/1  "<SPN530_EngineSpeedAtPoint4>"
  Bus Selector/6 -> Data Type Conversion5/1  "<SPN541_EnginePercentTorqueAtPoint3>"
  Bus Selector/5 -> Data Type Conversion4/1  "<SPN529_EngineSpeedAtPoint3>"
  Bus Selector/4 -> Data Type Conversion3/1  "<SPN540_EnginePercentTorqueAtPoint2>"
  Bus Selector/3 -> Data Type Conversion2/1  "<SPN528_EngineSpeedAtPoint2>"
  Bus Selector/2 -> Data Type Conversion1/1  "<SPN539_EnginePercentTorqueAtIdlePoint1>"
  Bus Selector/12 -> Data Type Conversion11/1  "<SPN545_EngineGainKpOfTheEndspeedGovernor>"
  Bus Selector/1 -> Data Type Conversion/1  "<SPN188_EngineSpeedAtIdlePoint1>"
  Data/1 -> Bus Selector/1

== system SUB_ECU_L4_MABX_HW_Interface_PIC_PB/INPUTS_PIC_PB/CAN_PIC_PB/Arb_PropB_REAX_3 ==
  Data : Inport
  Bus Selector : BusSelector  OutputSignals=Signals.PropB_REAX_3_CurrentOperatingMode,Signals.PropB_REAX_3_ReqOperatingMode,Signals.PropB_REAX_3_StatusErrMsg,Signals.PropB_REAX_3_HandwheelTorque,Signals.PropB_REAX_3_HandwheelVelocity,Signals.PropB_REAX_3_PullCompensation
  Data Type Conversion{,1..5} (6 alike) : DataTypeConversion  SaturateOnIntegerOverflow=on
  Terminator{,1..5} (6 alike) : Terminator
      settings: InitFcn=|
      | try
      |    MBDS_BlockCallback('Update', gcb);
      | end
  wires:
  Data Type Conversion5/1 -> Terminator5/1  "REAX_Pull_Compensation"
  Data Type Conversion4/1 -> Terminator4/1  "REAX_Handwheel_Velocity"
  Data Type Conversion3/1 -> Terminator3/1  "REAX_Handwheel_Torque"
  Data Type Conversion2/1 -> Terminator2/1  "REAX_Status"
  Data Type Conversion1/1 -> Terminator1/1  "REAX_Req_Mode"
  Data Type Conversion/1 -> Terminator/1  "REAX_Current_Mode"
  Bus Selector/6 -> Data Type Conversion5/1  "<PropB_REAX_3_PullCompensation>"
  Bus Selector/5 -> Data Type Conversion4/1  "<PropB_REAX_3_HandwheelVelocity>"
  Bus Selector/1 -> Data Type Conversion/1  "<PropB_REAX_3_CurrentOperatingMode>"
  Bus Selector/3 -> Data Type Conversion2/1  "<PropB_REAX_3_StatusErrMsg>"
  Bus Selector/4 -> Data Type Conversion3/1  "<PropB_REAX_3_HandwheelTorque>"
  Bus Selector/2 -> Data Type Conversion1/1  "<PropB_REAX_3_ReqOperatingMode>"
  Data/1 -> Bus Selector/1

== system SUB_ECU_L4_MABX_HW_Interface_PIC_PB/INPUTS_PIC_PB/CAN_PIC_PB/Arb_PropB_REAX_4 ==
  Data : Inport
  Bus Selector : BusSelector  OutputSignals=Signals.PropB_REAX_4_AbsSteeringPosValid,Signals.PropB_REAX_4_PositionIndexValid,Signals.PropB_REAX_4_DriverControlledEffortsEnabled,Signals.PropB_REAX_4_ControlOperatingMode,Signals.PropB_REAX_4_SystemMode,Signals.PropB_REAX_4_PercHandwheelTorque,Signals.PropB_REAX_4_AbsSteeringAngle,Signals.PropB_REAX_4_PercMotorTorque
  Data Type Conversion{,1..7} (8 alike) : DataTypeConversion  SaturateOnIntegerOverflow=on
  Terminator{,1..7} (8 alike) : Terminator
      settings: InitFcn=|
      | try
      |    MBDS_BlockCallback('Update', gcb);
      | end
  wires:
  Data Type Conversion7/1 -> Terminator7/1
  Data Type Conversion6/1 -> Terminator6/1
  Data Type Conversion5/1 -> Terminator5/1
  Data Type Conversion4/1 -> Terminator4/1
  Data Type Conversion3/1 -> Terminator3/1
  Data Type Conversion2/1 -> Terminator2/1
  Data Type Conversion/1 -> Terminator1/1
  Data Type Conversion1/1 -> Terminator/1
  Bus Selector/8 -> Data Type Conversion7/1  "<PropB_REAX_4_PercMotorTorque>"
  Bus Selector/7 -> Data Type Conversion6/1  "<PropB_REAX_4_AbsSteeringAngle>"
  Bus Selector/6 -> Data Type Conversion5/1  "<PropB_REAX_4_PercHandwheelTorque>"
  Bus Selector/1 -> Data Type Conversion1/1  "<PropB_REAX_4_AbsSteeringPosValid>"
  Bus Selector/2 -> Data Type Conversion/1  "<PropB_REAX_4_PositionIndexValid>"
  Bus Selector/5 -> Data Type Conversion4/1  "<PropB_REAX_4_SystemMode>"
  Bus Selector/3 -> Data Type Conversion2/1  "<PropB_REAX_4_DriverControlledEffortsEnabled>"
  Bus Selector/4 -> Data Type Conversion3/1  "<PropB_REAX_4_ControlOperatingMode>"
  Data/1 -> Bus Selector/1

== system SUB_ECU_L4_MABX_HW_Interface_PIC_PB/INPUTS_PIC_PB/CAN_PIC_PB/CAN1_RX_TPCM_FF_00 ==
  Constant : Constant  Value=ENUM_CAN_RX_T.RX_CAN_1
  Multiport_Switch : MultiPortSwitch  DataPortOrder=Specify indices  DataPortIndices={ENUM_CAN_RX_T.RX_CAN_1, ENUM_CAN_RX_T.RX_CAN_2, ENUM_CAN_RX_T.RX_CAN_3, ENUM_CAN_RX_T.RX_CAN_4, ENUM_CAN_RX_T.RX_CAN_5, ENUM_CAN_RX_T.RX_CAN_6}  DataPortForDefault=Additional data port  SaturateOnIntegerOverflow=on  InputSameDT=on
      settings: AttributesFormatString=Zero-based indexing: %<zeroidx>
  RX_CAN_1 : Subsystem
  SelectChannel : Subsystem
  Terminator{,1..4} (5 alike) : Terminator
      settings: InitFcn=|
      | try
      |    MBDS_BlockCallback('Update', gcb);
      | end
  TPCM_FF_00 : Outport
  wires:
  Constant/1 -> SelectChannel/1(In1), Multiport_Switch/1
  SelectChannel/1(CAN1) -> RX_CAN_1/1(Enable)
  RX_CAN_1/1(TPCM_FF_00) -> Multiport_Switch/8, Multiport_Switch/7, Multiport_Switch/6, Multiport_Switch/5, Multiport_Switch/4, Multiport_Switch/3, Multiport_Switch/2
  SelectChannel/6(CAN6) -> Terminator4/1
  SelectChannel/5(CAN5) -> Terminator3/1
  SelectChannel/4(CAN4) -> Terminator2/1
  SelectChannel/3(CAN3) -> Terminator1/1
  SelectChannel/2(CAN2) -> Terminator/1
  Multiport_Switch/1 -> TPCM_FF_00/1

== system SUB_ECU_L4_MABX_HW_Interface_PIC_PB/INPUTS_PIC_PB/CAN_PIC_PB/CAN1_RX_TPDT_FF_00 ==
  Constant : Constant  Value=ENUM_CAN_RX_T.RX_CAN_1
  Multiport_Switch : MultiPortSwitch  DataPortOrder=Specify indices  DataPortIndices={ENUM_CAN_RX_T.RX_CAN_1, ENUM_CAN_RX_T.RX_CAN_2, ENUM_CAN_RX_T.RX_CAN_3, ENUM_CAN_RX_T.RX_CAN_4, ENUM_CAN_RX_T.RX_CAN_5, ENUM_CAN_RX_T.RX_CAN_6}  DataPortForDefault=Additional data port  SaturateOnIntegerOverflow=on  InputSameDT=on
      settings: AttributesFormatString=Zero-based indexing: %<zeroidx>
  RX_CAN_1 : Subsystem
  SelectChannel : Subsystem
  Terminator{,1..4} (5 alike) : Terminator
      settings: InitFcn=|
      | try
      |    MBDS_BlockCallback('Update', gcb);
      | end
  TPDT_FF_00 : Outport
  wires:
  Multiport_Switch/1 -> TPDT_FF_00/1
  SelectChannel/2(CAN2) -> Terminator/1
  SelectChannel/3(CAN3) -> Terminator1/1
  SelectChannel/4(CAN4) -> Terminator2/1
  SelectChannel/5(CAN5) -> Terminator3/1
  SelectChannel/6(CAN6) -> Terminator4/1
  RX_CAN_1/1(TPDT_FF_00) -> Multiport_Switch/2, Multiport_Switch/3, Multiport_Switch/4, Multiport_Switch/5, Multiport_Switch/6, Multiport_Switch/7, Multiport_Switch/8
  SelectChannel/1(CAN1) -> RX_CAN_1/1(Enable)
  Constant/1 -> Multiport_Switch/1, SelectChannel/1(In1)

== system SUB_ECU_L4_MABX_HW_Interface_PIC_PB/INPUTS_PIC_PB/CAN_PIC_PB/CAN_RX_ACC1_2A ==
  Constant : Constant  Value=boolean(1)
  RX_CAN_1 : Subsystem
  ACC1_2A : Outport
  wires:
  RX_CAN_1/1(ACC1_2A) -> ACC1_2A/1
  Constant/1 -> RX_CAN_1/1(Enable)

== system SUB_ECU_L4_MABX_HW_Interface_PIC_PB/INPUTS_PIC_PB/CAN_PIC_PB/CAN_RX_AEBS1_2A ==
  Constant : Constant  Value=boolean(1)
  RX_CAN_1 : Subsystem
  AEBS1_2A : Outport
  wires:
  Constant/1 -> RX_CAN_1/1(Enable)
  RX_CAN_1/1(AEBS1_2A) -> AEBS1_2A/1

== system SUB_ECU_L4_MABX_HW_Interface_PIC_PB/INPUTS_PIC_PB/CAN_PIC_PB/CAN_RX_AIR1_31 ==
  Constant : Constant  Value=boolean(1)
  RX_CAN_1 : Subsystem
  AIR1_31 : Outport
  wires:
  RX_CAN_1/1(AIR1_31) -> AIR1_31/1
  Constant/1 -> RX_CAN_1/1(Enable)

== system SUB_ECU_L4_MABX_HW_Interface_PIC_PB/INPUTS_PIC_PB/CAN_PIC_PB/CAN_RX_AMB_00 ==
  Constant : Constant  Value=boolean(1)
  RX_CAN_1 : Subsystem
  AMB_00 : Outport
  wires:
  Constant/1 -> RX_CAN_1/1(Enable)
  RX_CAN_1/1(AMB_00) -> AMB_00/1

== system SUB_ECU_L4_MABX_HW_Interface_PIC_PB/INPUTS_PIC_PB/CAN_PIC_PB/CAN_RX_B2_31 ==
  Constant : Constant
  RX_CAN_4 : Subsystem
  B2_00 : Outport
  wires:
  RX_CAN_4/1(B2_31) -> B2_00/1
  Constant/1 -> RX_CAN_4/1(Enable)

== system SUB_ECU_L4_MABX_HW_Interface_PIC_PB/INPUTS_PIC_PB/CAN_PIC_PB/CAN_RX_Bendix_RADAR_Tracks ==
  Constant : Constant  Value=boolean(0)
  RX_CAN_1 : Subsystem
  Bendix_RADAR_Tracks : Outport
  wires:
  RX_CAN_1/1(Bendix_RADAR_Tracks) -> Bendix_RADAR_Tracks/1
  Constant/1 -> RX_CAN_1/1(Enable)

== system SUB_ECU_L4_MABX_HW_Interface_PIC_PB/INPUTS_PIC_PB/CAN_PIC_PB/CAN_RX_CCVS1_00 ==
  Constant : Constant  Value=boolean(1)
  RX_CAN_1 : Subsystem
  CCVS1_0 : Outport
  wires:
  Constant/1 -> RX_CAN_1/1(Enable)
  RX_CAN_1/1(CCVS1_0) -> CCVS1_0/1

== system SUB_ECU_L4_MABX_HW_Interface_PIC_PB/INPUTS_PIC_PB/CAN_PIC_PB/CAN_RX_CCVS1_31 ==
  Constant : Constant  Value=boolean(1)
  RX_CAN_1 : Subsystem
  CCVS1_31 : Outport
  wires:
  Constant/1 -> RX_CAN_1/1(Enable)
  RX_CAN_1/1(CCVS1_31_) -> CCVS1_31/1

== system SUB_ECU_L4_MABX_HW_Interface_PIC_PB/INPUTS_PIC_PB/CAN_PIC_PB/CAN_RX_COGSOGRapidUpdate_01 ==
  Constant : Constant
  RX_CAN_4 : Subsystem
  COGSOGRapidUpdate_01 : Outport
  wires:
  Constant/1 -> RX_CAN_4/1(Enable)
  RX_CAN_4/1(COGSOGRapidUpdate_01) -> COGSOGRapidUpdate_01/1

== system SUB_ECU_L4_MABX_HW_Interface_PIC_PB/INPUTS_PIC_PB/CAN_PIC_PB/CAN_RX_CVW_0B ==
  Constant : Constant  Value=boolean(1)
  RX_CAN_1 : Subsystem
  CVW_0B : Outport
  wires:
  Constant/1 -> RX_CAN_1/1(Enable)
  RX_CAN_1/1(CVW_0B) -> CVW_0B/1

== system SUB_ECU_L4_MABX_HW_Interface_PIC_PB/INPUTS_PIC_PB/CAN_PIC_PB/CAN_RX_EBC1_0B ==
  Constant1 : Constant  Value=boolean(1)
  RX_CAN_1_EBC1 : Subsystem
  EBC1_0B : Outport
  wires:
  Constant1/1 -> RX_CAN_1_EBC1/1(Enable)
  RX_CAN_1_EBC1/1(EBC1_0B_) -> EBC1_0B/1

== system SUB_ECU_L4_MABX_HW_Interface_PIC_PB/INPUTS_PIC_PB/CAN_PIC_PB/CAN_RX_EBC1_8B ==
  Constant1 : Constant  Value=boolean(1)
  RX_CAN_5_EBC1 : Subsystem
  EBC1_8B : Outport
  wires:
  RX_CAN_5_EBC1/1(EBC1_8B) -> EBC1_8B/1
  Constant1/1 -> RX_CAN_5_EBC1/1(Enable)

== system SUB_ECU_L4_MABX_HW_Interface_PIC_PB/INPUTS_PIC_PB/CAN_PIC_PB/CAN_RX_EBC2_0B ==
  Enable_RX_EBC2_0B : Constant  Value=boolean(1)
  RX_CAN_1 : Subsystem
  EBC2_0B : Outport
  wires:
  Enable_RX_EBC2_0B/1 -> RX_CAN_1/1(Enable)
  RX_CAN_1/1(EBC2_0B) -> EBC2_0B/1

== system SUB_ECU_L4_MABX_HW_Interface_PIC_PB/INPUTS_PIC_PB/CAN_PIC_PB/CAN_RX_EC1_00 ==
  TPCM_BAM_CAN1 : Inport
  TPDT_BAM_CAN1 : Inport  Port=2
  timeStamp : Inport  Port=3
  Bus Creator : BusCreator  Inputs=5
  Bus Selector13 : BusSelector  OutputSignals=RX_status
  Bus Selector5 : BusSelector  OutputSignals=Signals.TPCM_BAM.SPN2569_ParameterGroupNumber
  CAN_RX_EC1_00 : Subsystem  TreatAsAtomicUnit=on
  Constant2 : Constant  Value=uint32(hex2dec('FEE3'))
  Decode_EC1 : PTC_MBDS_LIB/J1939/Decoders/Decode_EC1  PTC_MBDS_BlockVersion=5.41  PTC_BlockType=PTC_MBDS_Decode_EC1
      settings: SourceProductName=PACCAR Technical Center MBDS Library
  EQ1 : PTC_MBDS_LIB/MBDS Standard Library/Basic Operations/Logic and Bit Operations/EQ  InputSameDT=on  PTC_MBDS_BlockVersion=5.41  PTC_BlockType=PTC_MBDS_EQ
      settings: SourceProductName=PACCAR Technical Center MBDS Library
  Logical Operator : Logic  AllPortsSameDT=off  OutDataTypeStr=boolean
  EC1_00 : Outport
  wires:
  timeStamp/1 -> CAN_RX_EC1_00/3(timeStamp)
  Logical Operator/1 -> CAN_RX_EC1_00/Enable
  Decode_EC1/1 -> [Signals]
  CAN_RX_EC1_00/2(RX_status) -> [RX_status]
  CAN_RX_EC1_00/4(RX_delta_time) -> [RX_delta_time]
  CAN_RX_EC1_00/3(RX_time) -> [RX_time]
  CAN_RX_EC1_00/1(RawData) -> Decode_EC1/1, [RawData]
  Bus Creator/1 -> EC1_00/1
  TPDT_BAM_CAN1/1 -> [TPDT_BAM_CAN1]
  [RX_delta_time] -> Bus Creator/5
  [RawData] -> Bus Creator/2
  [RX_status] -> Bus Creator/3
  [Signals] -> Bus Creator/1
  [RX_time] -> Bus Creator/4
  [TPDT_BAM_CAN1] -> CAN_RX_EC1_00/2(TPDT)
  [TPCM_BAM_CAN1] -> CAN_RX_EC1_00/1(TPCM)
  TPCM_BAM_CAN1/1 -> [TPCM_BAM_CAN1]
  Constant2/1 -> EQ1/2
  EQ1/1 -> Logical Operator/2
  [TPCM_BAM_CAN1] -> Bus Selector5/1
  Bus Selector5/1 -> EQ1/1  "<SPN2569_ParameterGroupNumber>"
  [TPDT_BAM_CAN1] -> Bus Selector13/1
  Bus Selector13/1 -> Logical Operator/1  "<RX_status>"

== system SUB_ECU_L4_MABX_HW_Interface_PIC_PB/INPUTS_PIC_PB/CAN_PIC_PB/CAN_RX_EEC1_00 ==
  Enable_RX_EEC1_00 : Constant  Value=boolean(1)
  RX_CAN_1 : Subsystem
  EEC1_00 : Outport
  wires:
  Enable_RX_EEC1_00/1 -> RX_CAN_1/1(Enable)
  RX_CAN_1/1(EEC1_00) -> EEC1_00/1

== system SUB_ECU_L4_MABX_HW_Interface_PIC_PB/INPUTS_PIC_PB/CAN_PIC_PB/CAN_RX_EEC2_00 ==
  Enable_RX_EEC2_00 : Constant  Value=boolean(1)
  RX_CAN_2 : Subsystem
  EEC2_00 : Outport
  wires:
  RX_CAN_2/1(EEC2_00) -> EEC2_00/1
  Enable_RX_EEC2_00/1 -> RX_CAN_2/1(Enable)

== system SUB_ECU_L4_MABX_HW_Interface_PIC_PB/INPUTS_PIC_PB/CAN_PIC_PB/CAN_RX_EEC3_00 ==
  Enable_RX_EEC3_00 : Constant  Value=boolean(1)
  RX_CAN_1 : Subsystem
  EEC3_00 : Outport
  wires:
  Enable_RX_EEC3_00/1 -> RX_CAN_1/1(Enable)
  RX_CAN_1/1(EEC3_00) -> EEC3_00/1
